simulink model "modelR2020a"  (R2020a)
settings: Solver=ode23s  StartTime=0.0  StopTime=settings.Tsim  FixedStep=0.1  RelTol=1e-6  AbsTol=1e-6
values from neighbouring files (symbols this model uses):
  settings = Simulink.Parameter    [main.m]
libraries: vrlib x5
settings Model: Creator=rosat  LastModifiedBy=rosat
settings SolverCC: ZeroCrossAlgorithm=Adaptive
settings OptimizationCC: BlockReduction=off  DefaultParameterBehavior=Inlined  BufferReuse=off
settings DebuggingCC: IgnoredZcDiagnostic=none  SFMachineParentedDataDiag=error

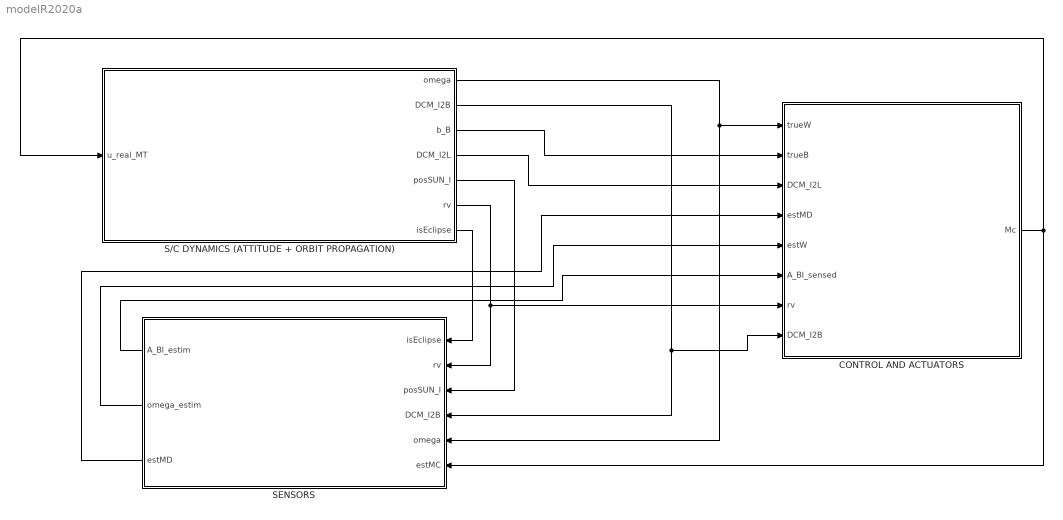
== system modelR2020a ==
  CONTROL AND ACTUATORS : Subsystem
  S/C DYNAMICS (ATTITUDE + ORBIT PROPAGATION) : Subsystem
  SENSORS : Subsystem
  wires:
  S/C DYNAMICS (ATTITUDE + ORBIT PROPAGATION)/3(b_B) -> CONTROL AND ACTUATORS/2(trueB)
  SENSORS/1(A_BI_estim) -> CONTROL AND ACTUATORS/6(A_BI_sensed)
  S/C DYNAMICS (ATTITUDE + ORBIT PROPAGATION)/6(rv) -> CONTROL AND ACTUATORS/7(rv), SENSORS/2(rv)
  SENSORS/3(estMD) -> CONTROL AND ACTUATORS/4(estMD)
  SENSORS/2(omega_estim) -> CONTROL AND ACTUATORS/5(estW)
  S/C DYNAMICS (ATTITUDE + ORBIT PROPAGATION)/2(DCM_I2B) -> CONTROL AND ACTUATORS/8(DCM_I2B), SENSORS/4(DCM_I2B)
  S/C DYNAMICS (ATTITUDE + ORBIT PROPAGATION)/1(omega) -> CONTROL AND ACTUATORS/1(trueW), SENSORS/5(omega)
  S/C DYNAMICS (ATTITUDE + ORBIT PROPAGATION)/4(DCM_I2L) -> CONTROL AND ACTUATORS/3(DCM_I2L)
  S/C DYNAMICS (ATTITUDE + ORBIT PROPAGATION)/5(posSUN_I) -> SENSORS/3(posSUN_I)
  CONTROL AND ACTUATORS/1(Mc) -> S/C DYNAMICS (ATTITUDE + ORBIT PROPAGATION)/1(u_real_MT), SENSORS/6(estMC)
  S/C DYNAMICS (ATTITUDE + ORBIT PROPAGATION)/7(isEclipse) -> SENSORS/1(isEclipse)

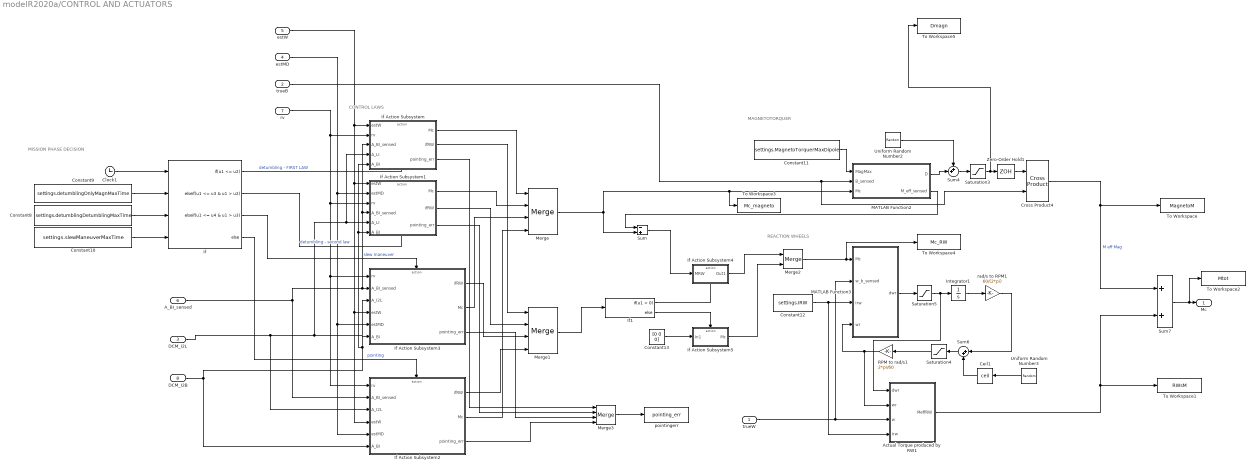
== system modelR2020a/CONTROL AND ACTUATORS ==
  note: REACTION WHEELS
  note: CONTROL LAWS
  note: MISSION PHASE DECISION
  note: MAGNETOTORQUER
  trueW : Inport
  trueB : Inport  Port=2
  DCM_I2L : Inport  Port=3
  estMD : Inport  Port=4
  estW : Inport  Port=5
  A_BI_sensed : Inport  Port=6
  rv : Inport  Port=7
  DCM_I2B : Inport  Port=8
  Actual Torque produced by RW1 : MATLAB Function  TreatAsAtomicUnit=on
  Ceil1 : Rounding  Operator=ceil
  Clock1 : Clock
  Constant10 : Constant  Value=settings.slewManeuverMaxTime
  Constant11 : Constant  Value=settings.MagnetoTorquerMaxDipole
  Constant12 : Constant  Value=settings.IRW
  Constant13 : Constant  Value=[0 0 0]
  Constant8 : Constant  Value=settings.detumblingDetumblingMaxTime
  Constant9 : Constant  Value=settings.detumblingOnlyMagnMaxTime
  Cross Product4 : vrlib/Utilities/Cross Product
  If : If  NumInputs=4  IfExpression=u1 <= u2  ElseIfExpressions=u1 <= u3 & u1 > u2, u1 <= u4 & u1 > u3
  If Action Subsystem : Subsystem  TreatAsAtomicUnit=on
  If Action Subsystem1 : Subsystem  TreatAsAtomicUnit=on
  If Action Subsystem2 : Subsystem  TreatAsAtomicUnit=on
  If Action Subsystem3 : Subsystem  TreatAsAtomicUnit=on
  If Action Subsystem4 : Subsystem  TreatAsAtomicUnit=on
  If Action Subsystem5 : Subsystem  TreatAsAtomicUnit=on
  If1 : If
  Integrator1 : Integrator  InitialCondition=[0;0;0]
  MATLAB Function2 : MATLAB Function  TreatAsAtomicUnit=on
  MATLAB Function3 : MATLAB Function  TreatAsAtomicUnit=on
  Merge : Merge  Inputs=4
  Merge1 : Merge  Inputs=4
  Merge2 : Merge
  Merge3 : Merge  Inputs=4
  RPM to rad/s1 : Gain  Gain=2*pi/60
  Saturation3 : Saturate  UpperLimit=settings.MagnetoTorquerMaxDipole  LowerLimit=-settings.MagnetoTorquerMaxDipole
  Saturation4 : Saturate  UpperLimit=settings.MaxRPM*[1;1;1]  LowerLimit=-settings.MaxRPM*[1;1;1]  LinearizeAsGain=off  ZeroCross=off
  Saturation5 : Saturate  UpperLimit=settings.MaxRPM_Rate  LowerLimit=-settings.MaxRPM_Rate
  Sum : Sum  Inputs=-+
  Sum4 : Sum  Inputs=++|
  Sum6 : Sum  Inputs=|++
  Sum7 : Sum
  To Workspace : ToWorkspace  VariableName=MagnetoM  SaveFormat=Timeseries  SampleTime=-1
  To Workspace1 : ToWorkspace  VariableName=RWsM  SaveFormat=Timeseries  SampleTime=-1
  To Workspace2 : ToWorkspace  VariableName=Mtot  SaveFormat=Timeseries  SampleTime=-1
  To Workspace3 : ToWorkspace  VariableName=Mc_magneto  SaveFormat=Timeseries  SampleTime=-1
  To Workspace4 : ToWorkspace  VariableName=Mc_RW  SaveFormat=Timeseries  SampleTime=-1
  To Workspace5 : ToWorkspace  VariableName=Dmagn  SaveFormat=Timeseries  SampleTime=-1
  Uniform Random Number2 : UniformRandomNumber  Minimum=-settings.MagnetoTorquerDipoleError*[1;1;1]  Maximum=settings.MagnetoTorquerDipoleError*[1;1;1]  Seed=456156  SampleTime=1/settings.MagnetoTorquerSampleRate
  Uniform Random Number3 : UniformRandomNumber  Minimum=-settings.RPMAccuracy*[1;1;1]  Maximum=settings.RPMAccuracy*[1;1;1]  Seed=561651  SampleTime=1/settings.RW_sr
  Zero-Order Hold1 : ZeroOrderHold  SampleTime=1/settings.MagnetoTorquerSampleRate
  pointingerr : ToWorkspace  VariableName=pointing_err  SaveFormat=Timeseries  SampleTime=-1
  rad/s to RPM1 : Gain  Gain=60/(2*pi)
  Mc : Outport
  wires:
  Clock1/1 -> If/1
  Constant9/1 -> If/2
  Constant8/1 -> If/3
  If/1 -> If Action Subsystem/Action  "detumbling - FIRST LAW"
  If/2 -> If Action Subsystem1/Action  "detumbling - second law"
  If/4 -> If Action Subsystem2/Action  "pointing"
  Constant10/1 -> If/4
  If/3 -> If Action Subsystem3/Action  "slew maneuver"
  Sum4/1 -> Saturation3/1
  Zero-Order Hold1/1 -> Cross Product4/1
  Constant11/1 -> MATLAB Function2/1(MagMax)
  Saturation3/1 -> To Workspace5/1, Zero-Order Hold1/1
  Uniform Random Number2/1 -> Sum4/1
  If Action Subsystem/1(Mc) -> Merge/1
  If Action Subsystem1/1(Mc) -> Merge/2
  If Action Subsystem/2(ifRW) -> Merge1/1
  If Action Subsystem1/2(ifRW) -> Merge1/2
  If Action Subsystem3/2(Mc) -> Merge/3
  If Action Subsystem3/1(ifRW) -> Merge1/3
  Cross Product4/1 -> To Workspace/1, Sum7/1  "M eff Mag"
  rad/s to RPM1/1 -> Sum6/1
  Uniform Random Number3/1 -> Ceil1/1
  RPM to rad/s1/1 -> Actual Torque produced by RW1/2(wr), MATLAB Function3/4(wr)
  Constant12/1 -> Actual Torque produced by RW1/4(Irw), MATLAB Function3/3(Irw)
  MATLAB Function3/1(dwr) -> Saturation5/1
  Saturation4/1 -> RPM to rad/s1/1
  Sum6/1 -> Saturation4/1
  Integrator1/1 -> rad/s to RPM1/1
  Saturation5/1 -> Actual Torque produced by RW1/1(dwr), Integrator1/1
  If1/1 -> If Action Subsystem4/Action
  If1/2 -> If Action Subsystem5/Action
  Constant13/1 -> If Action Subsystem5/1(In1)
  Merge2/1 -> To Workspace4/1, MATLAB Function3/1(Mc)
  If Action Subsystem4/1(Out1) -> Merge2/1
  If Action Subsystem5/1(Mc) -> Merge2/2
  Sum7/1 -> To Workspace2/1, Mc/1
  Actual Torque produced by RW1/1(MeffRW) -> To Workspace1/1, Sum7/2
  MATLAB Function2/1(D) -> Sum4/2
  Merge1/1 -> If1/1
  Sum/1 -> If Action Subsystem4/1(MRW)
  Ceil1/1 -> Sum6/2
  MATLAB Function2/2(M_eff_sensed) -> Sum/1
  Merge/1 -> To Workspace3/1, MATLAB Function2/3(Mc), Sum/2
  estW/1 -> If Action Subsystem2/4(estW), If Action Subsystem3/4(estW), If Action Subsystem1/1(estW), If Action Subsystem/1(estW)
  trueW/1 -> Actual Torque produced by RW1/3(w), MATLAB Function3/2(w_b_sensed)
  estMD/1 -> If Action Subsystem2/5(estMD), If Action Subsystem3/5(estMD), If Action Subsystem1/2(estMD)
  trueB/1 -> Cross Product4/2, MATLAB Function2/2(B_sensed)
  rv/1 -> If Action Subsystem/2(rv), If Action Subsystem1/3(rv), If Action Subsystem2/1(rv), If Action Subsystem3/1(rv)
  A_BI_sensed/1 -> If Action Subsystem1/4(A_BI_sensed), If Action Subsystem/3(A_BI_sensed), If Action Subsystem3/2(A_BI_sensed), If Action Subsystem2/2(A_BI_sensed)
  DCM_I2B/1 -> If Action Subsystem1/6(A_BI), If Action Subsystem/5(A_BI), If Action Subsystem3/6(A_BI), If Action Subsystem2/6(A_BI)
  DCM_I2L/1 -> If Action Subsystem3/3(A_I2L), If Action Subsystem1/5(A_LI), If Action Subsystem/4(A_LI), If Action Subsystem2/3(A_I2L)
  If Action Subsystem2/2(Mc) -> Merge/4
  If Action Subsystem2/1(ifRW) -> Merge1/4
  If Action Subsystem/3(pointing_err) -> Merge3/1
  If Action Subsystem1/3(pointing_err) -> Merge3/2
  If Action Subsystem3/3(pointing_err) -> Merge3/3
  If Action Subsystem2/3(pointing_err) -> Merge3/4
  Merge3/1 -> pointingerr/1

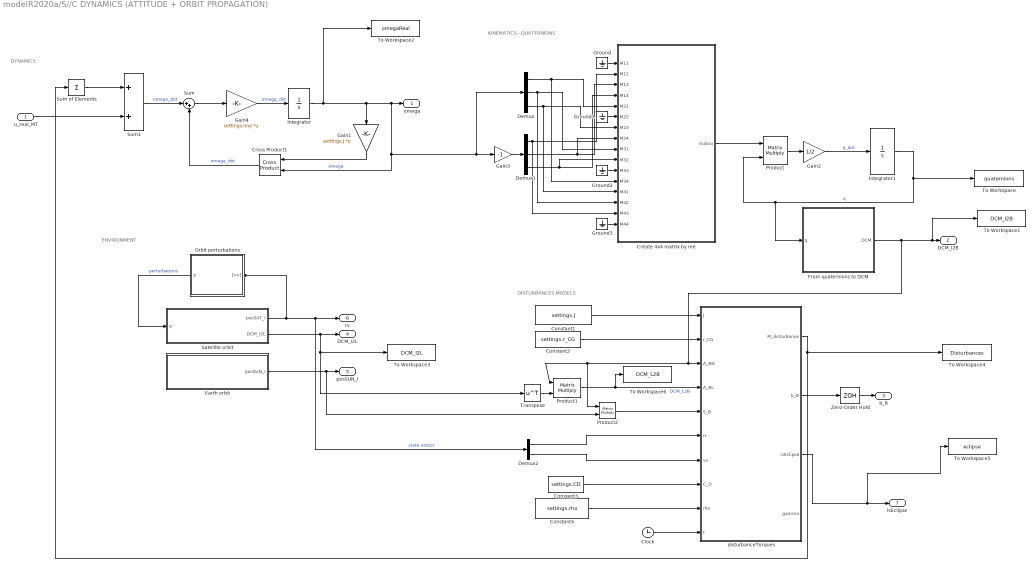
== system modelR2020a/S//C DYNAMICS (ATTITUDE + ORBIT PROPAGATION) ==
  note: DISTURBANCES MODELS
  note: ENVIRONMENT
  note: KINEMATICS - QUATERNIONS
  note: DYNAMICS
  u_real_MT : Inport
  Clock : Clock
  Constant1 : Constant  Value=settings.J
  Constant2 : Constant  Value=settings.r_CG
  Constant3 : Constant  Value=settings.CD
  Constant4 : Constant  Value=settings.rho
  Create 4x4 matrix by me : Subsystem
  Cross Product1 : vrlib/Utilities/Cross Product
  Demux : Demux  Outputs=3
  Demux1 : Demux  Outputs=3
  Demux2 : Demux  Outputs=2
  Earth orbit : Subsystem
  From quaternions to DCM : Subsystem
  Gain1 : Gain  Gain=settings.J  Multiplication=Matrix(K*u)
  Gain2 : Gain  Gain=1/2
  Gain3 : Gain  Gain=-1
  Gain4 : Gain  Gain=settings.invJ  Multiplication=Matrix(K*u)
  Ground{,1..3} (4 alike) : Ground
  Integrator : Integrator  InitialCondition=settings.omega0
  Integrator1 : Integrator  InitialCondition=settings.q0
  Orbit perturbations : Subsystem
  Product : Product  Multiplication=Matrix(*)
  Product1 : Product  Multiplication=Matrix(*)
  Product2 : Product  Multiplication=Matrix(*)
  Satellite orbit : Subsystem
  Sum : Sum  Inputs=|++
  Sum of Elements : Sum  Inputs=+  CollapseMode=Specified dimension  CollapseDim=2
  Sum1 : Sum
  To Workspace : ToWorkspace  VariableName=quaternions  SaveFormat=Timeseries  SampleTime=-1
  To Workspace1 : ToWorkspace  VariableName=DCM_I2B  SaveFormat=Timeseries  SampleTime=-1
  To Workspace2 : ToWorkspace  VariableName=omegaReal  SaveFormat=Timeseries  SampleTime=-1
  To Workspace3 : ToWorkspace  VariableName=DCM_I2L  SaveFormat=Timeseries  SampleTime=-1
  To Workspace4 : ToWorkspace  VariableName=Disturbances  SaveFormat=Timeseries  SampleTime=-1
  To Workspace5 : ToWorkspace  VariableName=eclipse  SaveFormat=Timeseries  SampleTime=-1
  To Workspace6 : ToWorkspace  VariableName=DCM_L2B  SaveFormat=Timeseries  SampleTime=-1
  Transpose : Math  Operator=transpose  SaturateOnIntegerOverflow=on
  Zero-Order Hold : ZeroOrderHold  SampleTime=0.01
  disturbanceTorques : MATLAB Function  TreatAsAtomicUnit=on
  omega : Outport
  DCM_I2B : Outport  Port=2
  b_B : Outport  Port=3
  DCM_I2L : Outport  Port=4
  posSUN_I : Outport  Port=5
  rv : Outport  Port=6
  isEclipse : Outport  Port=7
  wires:
  Sum of Elements/1 -> Sum1/1
  Integrator/1 -> Demux/1, Gain3/1, Cross Product1/2, omega/1, Gain1/1, To Workspace2/1  "omega"
  Sum/1 -> Gain4/1
  u_real_MT/1 -> Sum1/2
  Sum1/1 -> Sum/1  "omega_dot"
  Gain4/1 -> Integrator/1  "omega_dot"
  Cross Product1/1 -> Sum/2  "omega_dot"
  Gain1/1 -> Cross Product1/1
  disturbanceTorques/1(M_disturbance) -> To Workspace4/1, Sum of Elements/1
  Demux/3 -> Create 4x4 matrix by me/13(M41), Create 4x4 matrix by me/7(M23)
  Product/1 -> Gain2/1
  Demux1/2 -> Create 4x4 matrix by me/8(M24), Create 4x4 matrix by me/3(M13)
  Demux1/3 -> Create 4x4 matrix by me/10(M32), Create 4x4 matrix by me/4(M14)
  Demux1/1 -> Create 4x4 matrix by me/15(M43), Create 4x4 matrix by me/2(M12)
  Demux/1 -> Create 4x4 matrix by me/12(M34), Create 4x4 matrix by me/5(M21)
  Ground2/1 -> Create 4x4 matrix by me/11(M33)
  Ground/1 -> Create 4x4 matrix by me/1(M11)
  From quaternions to DCM/1(DCM) -> Product2/1, Product1/1, disturbanceTorques/3(A_BN), To Workspace1/1, DCM_I2B/1
  Demux/2 -> Create 4x4 matrix by me/14(M42), Create 4x4 matrix by me/9(M31)
  Ground3/1 -> Create 4x4 matrix by me/16(M44)
  Gain2/1 -> Integrator1/1  "q_dot"
  Integrator1/1 -> To Workspace/1, From quaternions to DCM/1(q), Product/2  "q"
  Gain3/1 -> Demux1/1
  Ground1/1 -> Create 4x4 matrix by me/6(M22)
  Create 4x4 matrix by me/1(matrix) -> Product/1
  Earth orbit/1(posSUN_I) -> Product2/2, posSUN_I/1
  Satellite orbit/1(posSAT_I) -> Orbit perturbations/1("[r;v]"), Demux2/1, rv/1  "state vector"
  Orbit perturbations/1(p) -> Satellite orbit/1(p)  "perturbations"
  Satellite orbit/2(DCM_I2L) -> Transpose/1, To Workspace3/1, DCM_I2L/1
  Constant3/1 -> disturbanceTorques/8(C_D)
  Constant2/1 -> disturbanceTorques/2(r_CG)
  Demux2/2 -> disturbanceTorques/7(vv)
  Demux2/1 -> disturbanceTorques/6(rr)
  Constant4/1 -> disturbanceTorques/9(rho)
  Clock/1 -> disturbanceTorques/10(t)
  Transpose/1 -> Product1/2
  Product2/1 -> disturbanceTorques/5(S_B)
  Product1/1 -> To Workspace6/1, disturbanceTorques/4(A_BL)  "DCM_L2B"
  Constant1/1 -> disturbanceTorques/1(J)
  disturbanceTorques/2(b_B) -> Zero-Order Hold/1
  Zero-Order Hold/1 -> b_B/1
  disturbanceTorques/3(isEclipse) -> To Workspace5/1, isEclipse/1

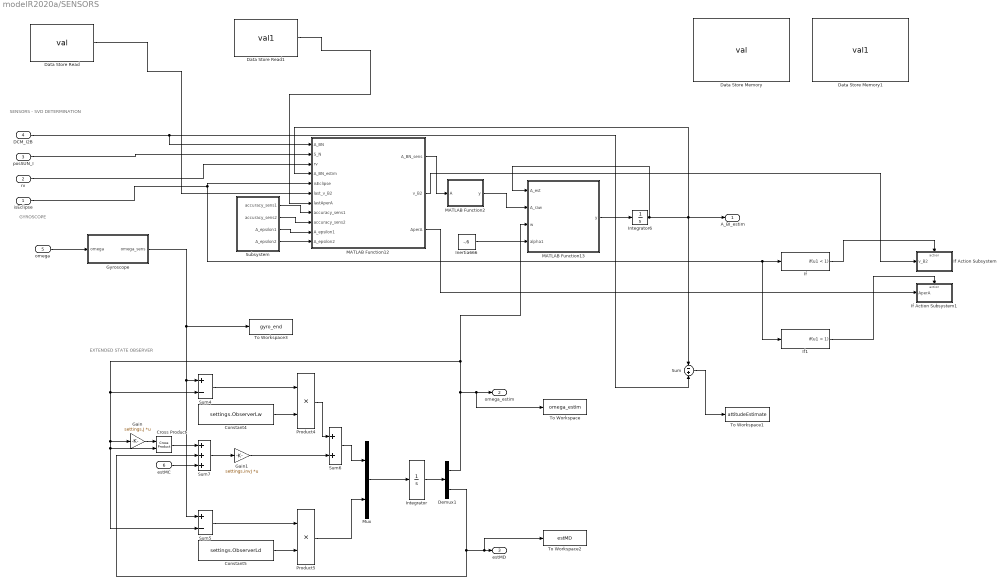
== system modelR2020a/SENSORS ==
  note: GYROSCOPE
  note: EXTENDED STATE OBSERVER
  note: SENSORS - SVD DETERMINATION
  isEclipse : Inport
  rv : Inport  Port=2
  posSUN_I : Inport  Port=3
  DCM_I2B : Inport  Port=4
  omega : Inport  Port=5
  estMC : Inport  Port=6
  Constant4 : Constant  Value=settings.ObserverLw
  Constant5 : Constant  Value=settings.ObserverLd
  Cross Product : vrlib/Utilities/Cross Product
  Data Store Memory : DataStoreMemory  DataStoreName=val  ReadBeforeWriteMsg=warning  WriteAfterWriteMsg=warning  WriteAfterReadMsg=warning  VectorParams1D=off  ShowAdditionalParam=off  Dimensions=3
  Data Store Memory1 : DataStoreMemory  DataStoreName=val1  ReadBeforeWriteMsg=warning  WriteAfterWriteMsg=warning  WriteAfterReadMsg=warning  VectorParams1D=off  ShowAdditionalParam=off  Dimensions=[3,3]
  Data Store Read : DataStoreRead  DataStoreName=val
  Data Store Read1 : DataStoreRead  DataStoreName=val1
  Demux1 : Demux  Outputs=2
  Gain : Gain  Gain=settings.J  Multiplication=Matrix(K*u)
  Gain1 : Gain  Gain=settings.invJ  Multiplication=Matrix(K*u)
  Gyroscope : Subsystem
  If : If  IfExpression=u1 < 1  ShowElse=off
  If Action Subsystem : Subsystem  TreatAsAtomicUnit=on
  If Action Subsystem1 : Subsystem  TreatAsAtomicUnit=on
  If1 : If  IfExpression=u1 < 1  ShowElse=off
  Inertia666 : Constant  Value=-.6
  Integrator : Integrator  InitialCondition=[settings.omega0; settings.ObserverMd0]
  Integrator6 : Integrator  InitialCondition=zeros(3,3)
  MATLAB Function12 : MATLAB Function  TreatAsAtomicUnit=on
  MATLAB Function13 : MATLAB Function  TreatAsAtomicUnit=on
  MATLAB Function2 : MATLAB Function  TreatAsAtomicUnit=on
  Mux : Mux  Inputs=2
  Product4 : Product
  Product5 : Product
  Subsystem : Subsystem
  Sum : Sum  Inputs=-+
  Sum4 : Sum  Inputs=+-
  Sum5 : Sum  Inputs=+-
  Sum6 : Sum
  Sum7 : Sum  Inputs=+++
  To Workspace : ToWorkspace  VariableName=omega_estim  SaveFormat=Timeseries  SampleTime=-1
  To Workspace1 : ToWorkspace  VariableName=attitudeEstimate  SaveFormat=Timeseries  SampleTime=-1
  To Workspace2 : ToWorkspace  VariableName=estMD  SaveFormat=Timeseries  SampleTime=-1
  To Workspace3 : ToWorkspace  VariableName=gyro_end  SaveFormat=Timeseries  SampleTime=-1
  A_BI_estim : Outport
  omega_estim : Outport  Port=2
  estMD : Outport  Port=3
  wires:
  DCM_I2B/1 -> Sum/2, MATLAB Function12/1(A_BN)
  posSUN_I/1 -> MATLAB Function12/2(S_N)
  omega/1 -> Gyroscope/1(omega)
  Gyroscope/1(omega_sens) -> To Workspace3/1, Sum5/1, Sum4/1
  Sum4/1 -> Product4/1
  Constant4/1 -> Product4/2
  Constant5/1 -> Product5/2
  Sum5/1 -> Product5/1
  Integrator/1 -> Demux1/1
  Demux1/1 -> MATLAB Function13/3(w), Sum5/2, Cross Product/2, Gain/1, Sum4/2, To Workspace/1, omega_estim/1
  Product4/1 -> Sum6/1
  Gain/1 -> Cross Product/1
  Cross Product/1 -> Sum7/1
  Demux1/2 -> To Workspace2/1, estMD/1, Sum7/2
  Sum7/1 -> Gain1/1
  Gain1/1 -> Sum6/2
  Sum6/1 -> Mux/1
  Product5/1 -> Mux/2
  Mux/1 -> Integrator/1
  estMC/1 -> Sum7/3
  Subsystem/1(accuracy_sens1) -> MATLAB Function12/8(accuracy_sens1)
  Subsystem/4(A_epsilon2) -> MATLAB Function12/11(A_epsilon2)
  MATLAB Function13/1(y) -> Integrator6/1
  MATLAB Function12/1(A_BN_sens) -> MATLAB Function2/1(A)
  Subsystem/3(A_epsilon1) -> MATLAB Function12/10(A_epsilon1)
  MATLAB Function2/1(y) -> MATLAB Function13/2(A_raw)
  Inertia666/1 -> MATLAB Function13/4(alpha1)
  Subsystem/2(accuracy_sens2) -> MATLAB Function12/9(accuracy_sens2)
  rv/1 -> MATLAB Function12/3(rv)
  Integrator6/1 -> A_BI_estim/1, MATLAB Function12/4(A_BN_estim), Sum/1, MATLAB Function13/1(A_est)
  isEclipse/1 -> If1/1, If/1, MATLAB Function12/5(isEclipse)
  MATLAB Function12/2(v_B2) -> If Action Subsystem/1(v_B2)
  If/1 -> If Action Subsystem/Action
  Data Store Read/1 -> MATLAB Function12/6(last_v_B2)
  MATLAB Function12/3(AperA) -> If Action Subsystem1/1(AperA)
  Data Store Read1/1 -> MATLAB Function12/7(lastAperA)
  If1/1 -> If Action Subsystem1/Action
  Sum/1 -> To Workspace1/1

== system modelR2020a/CONTROL AND ACTUATORS/If Action Subsystem ==
  estW : Inport
  rv : Inport  Port=2
  A_BI_sensed : Inport  Port=3
  A_LI : Inport  Port=4
  A_BI : Inport  Port=5
  Action Port : ActionPort  ActionPortLabel=if(u1 <= u2)
  Constant : Constant  Value=settings.detumblingkb
  Constant1 : Constant  Value=0
  Gain : Gain  Gain=-1
  MATLAB Function : MATLAB Function  TreatAsAtomicUnit=on
  Product : Product
  Mc : Outport
  ifRW : Outport  Port=2
  pointing_err : Outport  Port=3
  wires:
  Constant/1 -> Product/2
  Constant1/1 -> ifRW/1
  Product/1 -> Gain/1
  Gain/1 -> Mc/1
  A_BI_sensed/1 -> MATLAB Function/2(A_BI_sensed)
  MATLAB Function/3(pointing_err) -> pointing_err/1
  estW/1 -> MATLAB Function/4(estW), Product/1
  A_LI/1 -> MATLAB Function/3(A_LI)
  rv/1 -> MATLAB Function/1(rv)
  A_BI/1 -> MATLAB Function/5(A_BI)

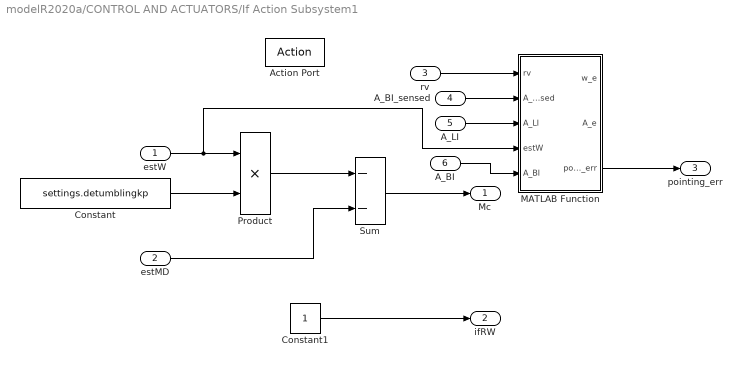
== system modelR2020a/CONTROL AND ACTUATORS/If Action Subsystem1 ==
  estW : Inport
  estMD : Inport  Port=2
  rv : Inport  Port=3
  A_BI_sensed : Inport  Port=4
  A_LI : Inport  Port=5
  A_BI : Inport  Port=6
  Action Port : ActionPort  ActionPortLabel=elseif(u1 <= u3 & u1 > u2)
  Constant : Constant  Value=settings.detumblingkp
  Constant1 : Constant
  MATLAB Function : MATLAB Function  TreatAsAtomicUnit=on
  Product : Product
  Sum : Sum  Inputs=--
  Mc : Outport
  ifRW : Outport  Port=2
  pointing_err : Outport  Port=3
  wires:
  estW/1 -> MATLAB Function/4(estW), Product/1
  Constant/1 -> Product/2
  Product/1 -> Sum/1
  estMD/1 -> Sum/2
  Sum/1 -> Mc/1
  Constant1/1 -> ifRW/1
  MATLAB Function/3(pointing_err) -> pointing_err/1
  rv/1 -> MATLAB Function/1(rv)
  A_BI_sensed/1 -> MATLAB Function/2(A_BI_sensed)
  A_LI/1 -> MATLAB Function/3(A_LI)
  A_BI/1 -> MATLAB Function/5(A_BI)

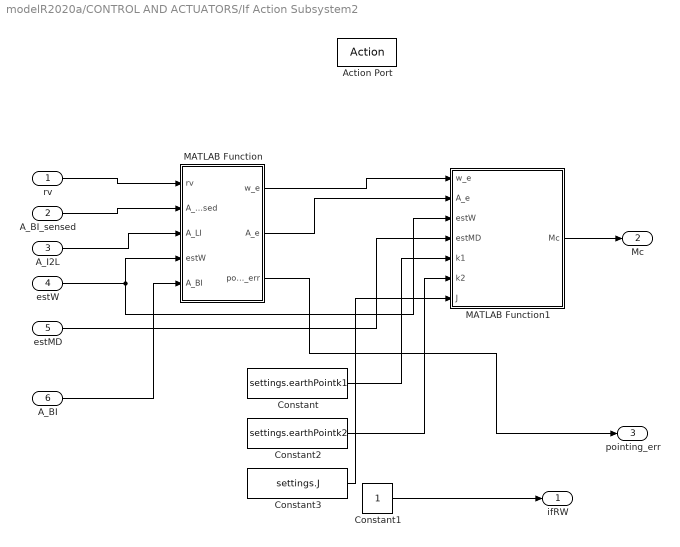
== system modelR2020a/CONTROL AND ACTUATORS/If Action Subsystem2 ==
  rv : Inport
  A_BI_sensed : Inport  Port=2
  A_I2L : Inport  Port=3
  estW : Inport  Port=4
  estMD : Inport  Port=5
  A_BI : Inport  Port=6
  Action Port : ActionPort  ActionPortLabel=else
  Constant : Constant  Value=settings.earthPointk1
  Constant1 : Constant
  Constant2 : Constant  Value=settings.earthPointk2
  Constant3 : Constant  Value=settings.J
  MATLAB Function : MATLAB Function  TreatAsAtomicUnit=on
  MATLAB Function1 : MATLAB Function  TreatAsAtomicUnit=on
  ifRW : Outport
  Mc : Outport  Port=2
  pointing_err : Outport  Port=3
  wires:
  A_BI/1 -> MATLAB Function/5(A_BI)
  estMD/1 -> MATLAB Function1/4(estMD)
  MATLAB Function/3(pointing_err) -> pointing_err/1
  rv/1 -> MATLAB Function/1(rv)
  Constant3/1 -> MATLAB Function1/7(J)
  A_BI_sensed/1 -> MATLAB Function/2(A_BI_sensed)
  A_I2L/1 -> MATLAB Function/3(A_LI)
  Constant2/1 -> MATLAB Function1/6(k2)
  estW/1 -> MATLAB Function1/3(estW), MATLAB Function/4(estW)
  Constant1/1 -> ifRW/1
  MATLAB Function1/1(Mc) -> Mc/1
  Constant/1 -> MATLAB Function1/5(k1)
  MATLAB Function/1(w_e) -> MATLAB Function1/1(w_e)
  MATLAB Function/2(A_e) -> MATLAB Function1/2(A_e)

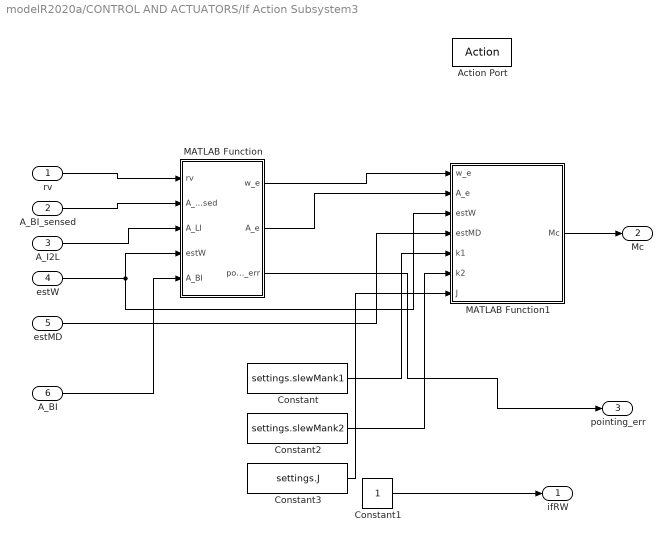
== system modelR2020a/CONTROL AND ACTUATORS/If Action Subsystem3 ==
  rv : Inport
  A_BI_sensed : Inport  Port=2
  A_I2L : Inport  Port=3
  estW : Inport  Port=4
  estMD : Inport  Port=5
  A_BI : Inport  Port=6
  Action Port : ActionPort  ActionPortLabel=elseif( u1 <= u4 & u1 > u3)
  Constant : Constant  Value=settings.slewMank1
  Constant1 : Constant
  Constant2 : Constant  Value=settings.slewMank2
  Constant3 : Constant  Value=settings.J
  MATLAB Function : MATLAB Function  TreatAsAtomicUnit=on
  MATLAB Function1 : MATLAB Function  TreatAsAtomicUnit=on
  ifRW : Outport
  Mc : Outport  Port=2
  pointing_err : Outport  Port=3
  wires:
  Constant1/1 -> ifRW/1
  rv/1 -> MATLAB Function/1(rv)
  estW/1 -> MATLAB Function1/3(estW), MATLAB Function/4(estW)
  A_I2L/1 -> MATLAB Function/3(A_LI)
  A_BI_sensed/1 -> MATLAB Function/2(A_BI_sensed)
  estMD/1 -> MATLAB Function1/4(estMD)
  MATLAB Function/1(w_e) -> MATLAB Function1/1(w_e)
  MATLAB Function/2(A_e) -> MATLAB Function1/2(A_e)
  MATLAB Function1/1(Mc) -> Mc/1
  Constant/1 -> MATLAB Function1/5(k1)
  Constant2/1 -> MATLAB Function1/6(k2)
  Constant3/1 -> MATLAB Function1/7(J)
  A_BI/1 -> MATLAB Function/5(A_BI)
  MATLAB Function/3(pointing_err) -> pointing_err/1

== system modelR2020a/CONTROL AND ACTUATORS/If Action Subsystem4 ==
  MRW : Inport
  Action Port : ActionPort  ActionPortLabel=if(u1 > 0)
  Out1 : Outport
  wires:
  MRW/1 -> Out1/1

== system modelR2020a/CONTROL AND ACTUATORS/If Action Subsystem5 ==
  In1 : Inport
  Action Port : ActionPort  ActionPortLabel=else
  Mc : Outport
  wires:
  In1/1 -> Mc/1

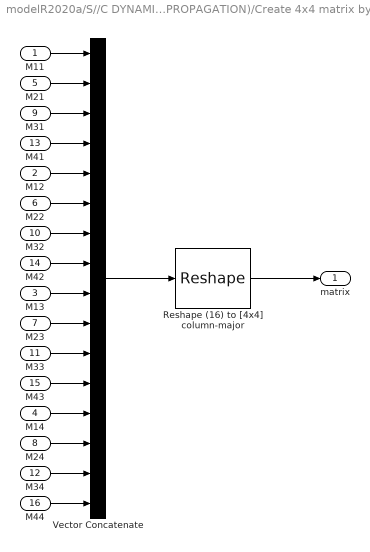
== system modelR2020a/S//C DYNAMICS (ATTITUDE + ORBIT PROPAGATION)/Create 4x4 matrix by me ==
  M11 : Inport
  M12 : Inport  Port=2
  M13 : Inport  Port=3
  M14 : Inport  Port=4
  M21 : Inport  Port=5
  M22 : Inport  Port=6
  M23 : Inport  Port=7
  M24 : Inport  Port=8
  M31 : Inport  Port=9
  M32 : Inport  Port=10
  M33 : Inport  Port=11
  M34 : Inport  Port=12
  M41 : Inport  Port=13
  M42 : Inport  Port=14
  M43 : Inport  Port=15
  M44 : Inport  Port=16
  Reshape (16) to [4x4] column-major : Reshape  OutputDimensionality=Customize  OutputDimensions=[4,4]
  Vector Concatenate : Concatenate  NumInputs=16
  matrix : Outport
  wires:
  M12/1 -> Vector Concatenate/5
  M11/1 -> Vector Concatenate/1
  M13/1 -> Vector Concatenate/9
  M14/1 -> Vector Concatenate/13
  M21/1 -> Vector Concatenate/2
  M44/1 -> Vector Concatenate/16
  M34/1 -> Vector Concatenate/15
  M24/1 -> Vector Concatenate/14
  M43/1 -> Vector Concatenate/12
  M33/1 -> Vector Concatenate/11
  M23/1 -> Vector Concatenate/10
  M42/1 -> Vector Concatenate/8
  M32/1 -> Vector Concatenate/7
  M22/1 -> Vector Concatenate/6
  M41/1 -> Vector Concatenate/4
  M31/1 -> Vector Concatenate/3
  Vector Concatenate/1 -> Reshape (16) to [4x4] column-major/1
  Reshape (16) to [4x4] column-major/1 -> matrix/1

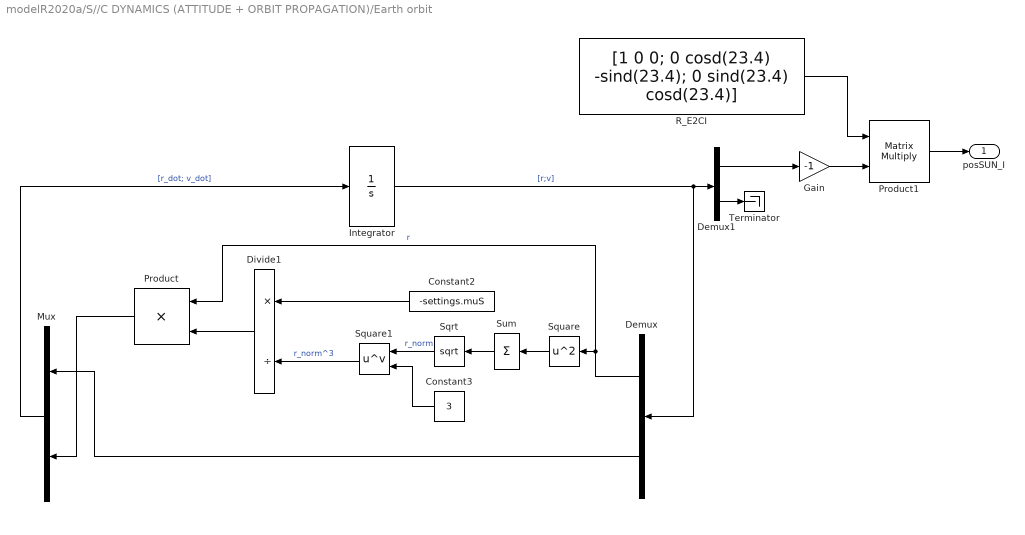
== system modelR2020a/S//C DYNAMICS (ATTITUDE + ORBIT PROPAGATION)/Earth orbit ==
  Constant2 : Constant  Value=-settings.muS
  Constant3 : Constant  Value=3
  Demux : Demux  Outputs=2
  Demux1 : Demux  Outputs=2
  Divide1 : Product  Inputs=*/
  Gain : Gain  Gain=-1
  Integrator : Integrator  InitialCondition=settings.Y0E
  Mux : Mux  Inputs=2
  Product : Product
  Product1 : Product  Multiplication=Matrix(*)
  R_E2CI : Constant  Value=[1 0 0; 0 cosd(23.4) -sind(23.4); 0 sind(23.4) cosd(23.4)]  VectorParams1D=off
  Sqrt : Sqrt  SaturateOnIntegerOverflow=on
  Square : Math  Operator=square  SaturateOnIntegerOverflow=on
  Square1 : Math  Operator=pow  SaturateOnIntegerOverflow=on
  Sum : Sum  Inputs=+
  Terminator : Terminator
  posSUN_I : Outport
  wires:
  Constant3/1 -> Square1/2
  Demux/1 -> Product/1, Square/1  "r"
  Demux/2 -> Mux/1
  Integrator/1 -> Demux1/1, Demux/1  "[r;v]"
  Divide1/1 -> Product/2
  Sqrt/1 -> Square1/1  "r_norm"
  Constant2/1 -> Divide1/1
  Product/1 -> Mux/2
  Sum/1 -> Sqrt/1
  Square/1 -> Sum/1
  Square1/1 -> Divide1/2  "r_norm^3"
  Mux/1 -> Integrator/1  "[r_dot; v_dot]"
  Gain/1 -> Product1/2
  R_E2CI/1 -> Product1/1
  Demux1/1 -> Gain/1
  Demux1/2 -> Terminator/1
  Product1/1 -> posSUN_I/1

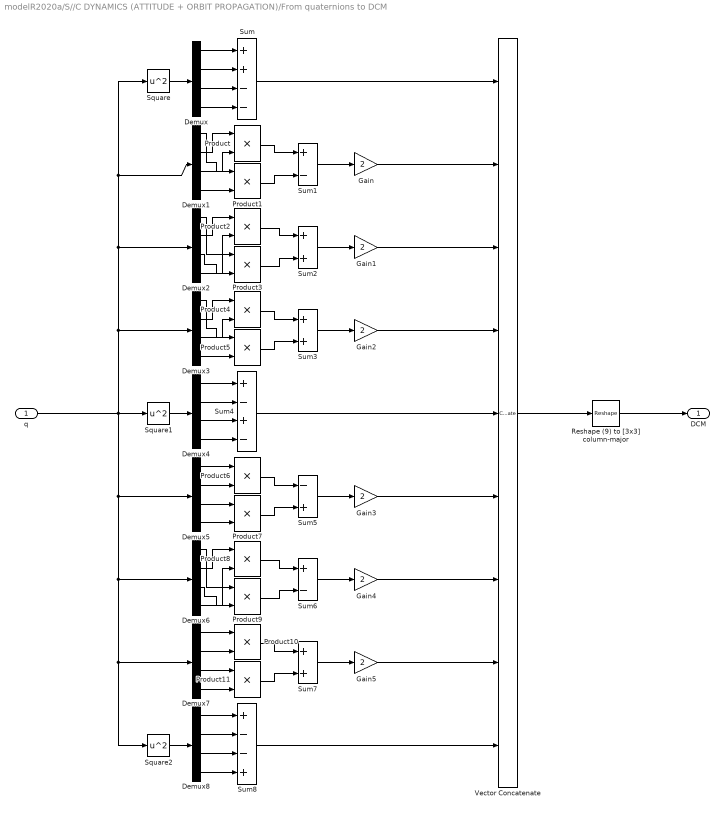
== system modelR2020a/S//C DYNAMICS (ATTITUDE + ORBIT PROPAGATION)/From quaternions to DCM ==
  q : Inport
  Demux{,1..8} (9 alike) : Demux
  Gain{,1..5} (6 alike) : Gain  Gain=2
  Product{,1..11} (12 alike) : Product
  Reshape (9) to [3x3] column-major : Reshape  OutputDimensionality=Customize  OutputDimensions=[3,3]
  Square : Math  Operator=square  SaturateOnIntegerOverflow=on
  Square1 : Math  Operator=square  SaturateOnIntegerOverflow=on
  Square2 : Math  Operator=square  SaturateOnIntegerOverflow=on
  Sum : Sum  Inputs=++--
  Sum1 : Sum  Inputs=+-
  Sum2 : Sum
  Sum3 : Sum
  Sum4 : Sum  Inputs=+-+-
  Sum5 : Sum  Inputs=-+
  Sum6 : Sum  Inputs=+-
  Sum7 : Sum
  Sum8 : Sum  Inputs=+--+
  Vector Concatenate : Concatenate  NumInputs=9
  DCM : Outport
  wires:
  q/1 -> Square/1, Demux1/1, Demux2/1, Demux3/1, Square1/1, Demux5/1, Demux6/1, Demux7/1, Square2/1
  Vector Concatenate/1 -> Reshape (9) to [3x3] column-major/1
  Square/1 -> Demux/1
  Demux/3 -> Sum/3
  Demux/4 -> Sum/4
  Demux/2 -> Sum/2
  Demux/1 -> Sum/1
  Sum/1 -> Vector Concatenate/1
  Demux1/2 -> Product/1
  Demux1/3 -> Product/2
  Demux1/1 -> Product1/1
  Demux1/4 -> Product1/2
  Product/1 -> Sum1/1
  Product1/1 -> Sum1/2
  Sum1/1 -> Gain/1
  Gain/1 -> Vector Concatenate/2
  Demux2/2 -> Product2/1
  Demux2/4 -> Product2/2
  Demux2/1 -> Product3/1
  Demux2/3 -> Product3/2
  Product3/1 -> Sum2/2
  Product2/1 -> Sum2/1
  Sum2/1 -> Gain1/1
  Gain1/1 -> Vector Concatenate/3
  Demux3/1 -> Product5/1
  Product5/1 -> Sum3/2
  Demux3/2 -> Product4/1
  Product4/1 -> Sum3/1
  Demux3/3 -> Product4/2
  Demux3/4 -> Product5/2
  Sum3/1 -> Gain2/1
  Gain2/1 -> Vector Concatenate/4
  Demux4/3 -> Sum4/3
  Demux4/1 -> Sum4/1
  Demux4/4 -> Sum4/4
  Sum4/1 -> Vector Concatenate/5
  Demux4/2 -> Sum4/2
  Square1/1 -> Demux4/1
  Product7/1 -> Sum5/2
  Product6/1 -> Sum5/1
  Sum5/1 -> Gain3/1
  Demux5/3 -> Product7/1
  Demux5/4 -> Product7/2
  Demux5/1 -> Product6/1
  Demux5/2 -> Product6/2
  Gain3/1 -> Vector Concatenate/6
  Sum6/1 -> Gain4/1
  Demux6/2 -> Product8/1
  Gain4/1 -> Vector Concatenate/7
  Demux6/4 -> Product8/2
  Demux6/3 -> Product9/2
  Demux6/1 -> Product9/1
  Product9/1 -> Sum6/2
  Product8/1 -> Sum6/1
  Demux7/2 -> Product10/2
  Demux7/3 -> Product11/1
  Sum7/1 -> Gain5/1
  Product10/1 -> Sum7/1
  Demux7/1 -> Product10/1
  Demux7/4 -> Product11/2
  Product11/1 -> Sum7/2
  Gain5/1 -> Vector Concatenate/8
  Demux8/2 -> Sum8/2
  Square2/1 -> Demux8/1
  Sum8/1 -> Vector Concatenate/9
  Demux8/3 -> Sum8/3
  Reshape (9) to [3x3] column-major/1 -> DCM/1
  Demux8/1 -> Sum8/1
  Demux8/4 -> Sum8/4

== system modelR2020a/S//C DYNAMICS (ATTITUDE + ORBIT PROPAGATION)/Orbit perturbations ==
  "[r;v]" : Inport
  Constant : Constant  Value=settings.orbitPert.J2
  If : If  IfExpression=u1
  J2 perturbation : Subsystem
  Terminator : Terminator
  if J2 perturbation : Subsystem  TreatAsAtomicUnit=on
  p : Outport
  wires:
  "[r;v]"/1 -> if J2 perturbation/1("[r;v]1")
  if J2 perturbation/1(Out1) -> J2 perturbation/1("[r;v]")
  J2 perturbation/1(p) -> p/1
  Constant/1 -> If/1
  If/2 -> Terminator/1
  If/1 -> if J2 perturbation/Action

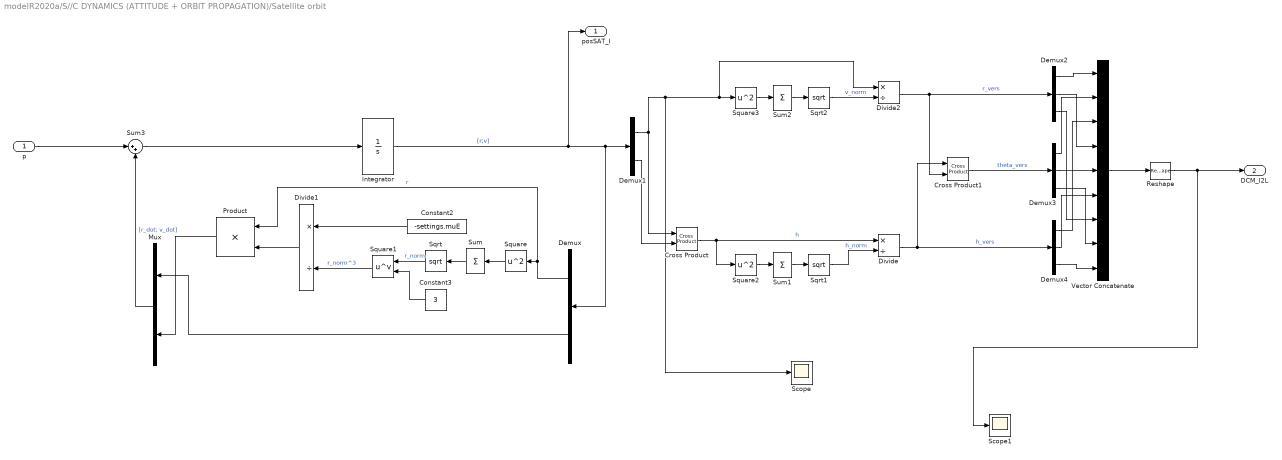
== system modelR2020a/S//C DYNAMICS (ATTITUDE + ORBIT PROPAGATION)/Satellite orbit ==
  p : Inport
  Constant2 : Constant  Value=-settings.muE
  Constant3 : Constant  Value=3
  Cross Product : vrlib/Utilities/Cross Product
  Cross Product1 : vrlib/Utilities/Cross Product
  Demux : Demux  Outputs=2
  Demux1 : Demux  Outputs=2
  Demux2 : Demux  Outputs=3
  Demux3 : Demux  Outputs=3
  Demux4 : Demux  Outputs=3
  Divide : Product  Inputs=*/
  Divide1 : Product  Inputs=*/
  Divide2 : Product  Inputs=*/
  Integrator : Integrator  InitialCondition=settings.Y0
  Mux : Mux  Inputs=2
  Product : Product
  Reshape : Reshape  OutputDimensionality=Customize  OutputDimensions=[3,3]
  Scope : Scope
  Scope1 : Scope
  Sqrt : Sqrt  SaturateOnIntegerOverflow=on
  Sqrt1 : Sqrt  SaturateOnIntegerOverflow=on
  Sqrt2 : Sqrt  SaturateOnIntegerOverflow=on
  Square : Math  Operator=square  SaturateOnIntegerOverflow=on
  Square1 : Math  Operator=pow  SaturateOnIntegerOverflow=on
  Square2 : Math  Operator=square  SaturateOnIntegerOverflow=on
  Square3 : Math  Operator=square  SaturateOnIntegerOverflow=on
  Sum : Sum  Inputs=+
  Sum1 : Sum  Inputs=+
  Sum2 : Sum  Inputs=+
  Sum3 : Sum  Inputs=|++
  Vector Concatenate : Concatenate  NumInputs=9
  posSAT_I : Outport
  DCM_I2L : Outport  Port=2
  wires:
  Constant3/1 -> Square1/2
  Demux/1 -> Product/1, Square/1  "r"
  Demux/2 -> Mux/1
  Integrator/1 -> Demux1/1, Demux/1, posSAT_I/1  "[r;v]"
  Divide1/1 -> Product/2
  Sqrt/1 -> Square1/1  "r_norm"
  Constant2/1 -> Divide1/1
  Product/1 -> Mux/2
  Sum/1 -> Sqrt/1
  Square/1 -> Sum/1
  Square1/1 -> Divide1/2  "r_norm^3"
  Mux/1 -> Sum3/2  "[r_dot; v_dot]"
  Sqrt2/1 -> Divide2/2  "v_norm"
  Divide2/1 -> Cross Product1/2, Demux2/1  "r_vers"
  Demux1/1 -> Cross Product/1, Scope/1, Divide2/1, Square3/1
  Demux2/2 -> Vector Concatenate/4
  Sqrt1/1 -> Divide/2  "h_norm"
  Demux4/1 -> Vector Concatenate/3
  Demux4/3 -> Vector Concatenate/9
  Demux3/3 -> Vector Concatenate/8
  Demux4/2 -> Vector Concatenate/6
  Vector Concatenate/1 -> Reshape/1
  Divide/1 -> Cross Product1/1, Demux4/1  "h_vers"
  Demux3/1 -> Vector Concatenate/2
  Sum1/1 -> Sqrt1/1
  Demux2/3 -> Vector Concatenate/7
  Square2/1 -> Sum1/1
  Demux2/1 -> Vector Concatenate/1
  Demux3/2 -> Vector Concatenate/5
  Cross Product/1 -> Divide/1, Square2/1  "h"
  Square3/1 -> Sum2/1
  Sum2/1 -> Sqrt2/1
  Cross Product1/1 -> Demux3/1  "theta_vers"
  Reshape/1 -> Scope1/1, DCM_I2L/1
  Demux1/2 -> Cross Product/2
  Sum3/1 -> Integrator/1
  p/1 -> Sum3/1

== system modelR2020a/SENSORS/Gyroscope ==
  omega : Inport
  ARW : RandomNumber  Variance=(1/4*deg2rad(settings.GyroscopeARW*[1;1;1]/sqrt(3600))).^2  Seed=1  SampleTime=1/settings.GyroscopeSampleRate
  Integrator : Integrator
  Integrator1 : Integrator  InitialCondition=[0 0 0 0 0 0]'
  MATLAB Function : MATLAB Function  TreatAsAtomicUnit=on
  MATLAB Function1 : MATLAB Function  TreatAsAtomicUnit=on
  RRW : RandomNumber  Variance=(1/4*deg2rad(settings.GyroscopeRRW*[1;1;1]/3600^3)).^2  Seed=2  SampleTime=1/settings.GyroscopeSampleRate
  Sum : Sum  Inputs=+++
  omega_sens : Outport
  wires:
  Sum/1 -> MATLAB Function/2(om)
  RRW/1 -> Integrator/1
  ARW/1 -> Sum/2
  Integrator/1 -> Sum/3
  omega/1 -> Sum/1
  MATLAB Function/1(x_dot) -> Integrator1/1
  Integrator1/1 -> MATLAB Function1/1(state_vector), MATLAB Function/1(x)
  MATLAB Function1/1(omega_raw) -> omega_sens/1

== system modelR2020a/SENSORS/If Action Subsystem ==
  v_B2 : Inport
  Action Port : ActionPort  ActionPortLabel=if(u1 < 1)
  Data Store Write : DataStoreWrite  DataStoreName=val
  wires:
  v_B2/1 -> Data Store Write/1

== system modelR2020a/SENSORS/If Action Subsystem1 ==
  AperA : Inport
  Action Port : ActionPort  ActionPortLabel=if(u1 < 1)
  Data Store Write : DataStoreWrite  DataStoreName=val1
  wires:
  AperA/1 -> Data Store Write/1

== system modelR2020a/SENSORS/Subsystem ==
  Earth Horizon : Constant  Value=settings.EarthSensorAccuracy
  MATLAB Function7 : MATLAB Function  TreatAsAtomicUnit=on
  Sun Sensor : Constant  Value=settings.SunSensorAccuracy
  err_EH : RandomNumber  Variance=(1/4*deg2rad(settings.EarthSensorAccuracy*[1 1 1])).^2  Seed=[1 2 3]  SampleTime=1/settings.EarthSensorSampleRate
  err_SS : RandomNumber  Variance=(1/4*deg2rad(settings.SunSensorAccuracy*[1 1 1])).^2  Seed=[4 5 6]  SampleTime=1/settings.SunSensorSampleRate
  accuracy_sens1 : Outport
  accuracy_sens2 : Outport  Port=2
  A_epsilon1 : Outport  Port=3
  A_epsilon2 : Outport  Port=4
  wires:
  MATLAB Function7/1(A_epsilon1) -> A_epsilon1/1
  MATLAB Function7/2(A_epsilon2) -> A_epsilon2/1
  Earth Horizon/1 -> accuracy_sens1/1
  Sun Sensor/1 -> accuracy_sens2/1
  err_SS/1 -> MATLAB Function7/2(accuracy_sens2)
  err_EH/1 -> MATLAB Function7/1(accuracy_sens1)

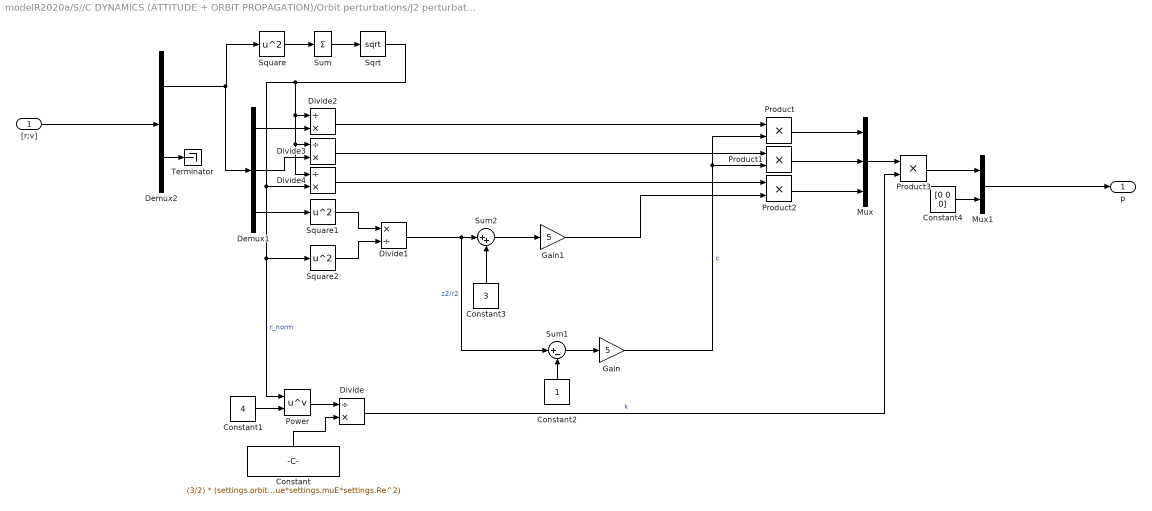
== system modelR2020a/S//C DYNAMICS (ATTITUDE + ORBIT PROPAGATION)/Orbit perturbations/J2 perturbation ==
  "[r;v]" : Inport
  Constant : Constant  Value=(3/2) * (settings.orbitPert.J2value*settings.muE*settings.Re^2)
  Constant1 : Constant  Value=4
  Constant2 : Constant
  Constant3 : Constant  Value=3
  Constant4 : Constant  Value=[0 0 0]
  Demux1 : Demux  Outputs=3
  Demux2 : Demux  Outputs=2
  Divide{,2..4} (4 alike) : Product  Inputs=/*
  Divide1 : Product  Inputs=*/
  Gain : Gain  Gain=5
  Gain1 : Gain  Gain=5
  Mux : Mux  Inputs=3
  Mux1 : Mux  Inputs=2
  Power : Math  Operator=pow  SaturateOnIntegerOverflow=on
  Product{,1..3} (4 alike) : Product
  Sqrt : Sqrt  SaturateOnIntegerOverflow=on
  Square : Math  Operator=square  SaturateOnIntegerOverflow=on
  Square1 : Math  Operator=square  SaturateOnIntegerOverflow=on
  Square2 : Math  Operator=square  SaturateOnIntegerOverflow=on
  Sum : Sum  Inputs=+
  Sum1 : Sum  Inputs=|+-
  Sum2 : Sum  Inputs=|++
  Terminator : Terminator
  p : Outport
  wires:
  "[r;v]"/1 -> Demux2/1
  Demux2/2 -> Terminator/1
  Square/1 -> Sum/1
  Sum/1 -> Sqrt/1
  Sqrt/1 -> Divide4/1, Divide3/1, Divide2/1, Divide4/2, Power/1, Square2/1  "r_norm"
  Demux2/1 -> Demux1/1, Square/1
  Constant/1 -> Divide/2
  Constant1/1 -> Power/2
  Power/1 -> Divide/1
  Demux1/3 -> Square1/1
  Square1/1 -> Divide1/1
  Square2/1 -> Divide1/2
  Constant2/1 -> Sum1/2
  Divide1/1 -> Sum1/1, Sum2/1  "z2/r2"
  Sum1/1 -> Gain/1
  Gain/1 -> Product1/2, Product/2  "c"
  Divide/1 -> Product3/2  "k"
  Demux1/1 -> Divide2/2
  Divide2/1 -> Product/1
  Demux1/2 -> Divide3/2
  Divide3/1 -> Product1/1
  Constant3/1 -> Sum2/2
  Sum2/1 -> Gain1/1
  Divide4/1 -> Product2/1
  Gain1/1 -> Product2/2
  Product/1 -> Mux/1
  Product1/1 -> Mux/2
  Product2/1 -> Mux/3
  Mux/1 -> Product3/1
  Product3/1 -> Mux1/1
  Constant4/1 -> Mux1/2
  Mux1/1 -> p/1

== system modelR2020a/S//C DYNAMICS (ATTITUDE + ORBIT PROPAGATION)/Orbit perturbations/if J2 perturbation ==
  "[r;v]1" : Inport
  Action Port : ActionPort  ActionPortLabel=if(u1)
  Out1 : Outport
  wires:
  "[r;v]1"/1 -> Out1/1

== matlab function modelR2020a/CONTROL AND ACTUATORS/MATLAB Function2 ==
  data: MagMax input; B_sensed input; Mc input; D output; M_eff_sensed output
function [D, M_eff_sensed] = fcn(MagMax,B_sensed,Mc)
D = cross(B_sensed, Mc)/norm(B_sensed);
if D(1)>MagMax
    D(1)=MagMax;
end
if D(2)>MagMax
    D(2)=MagMax;
end
if D(3)>MagMax
    D(3)=MagMax;
end
if D(1)<-MagMax
    D(1)=-MagMax;
end
if D(2)<-MagMax
    D(2)=-MagMax;
end
if D(3)<-MagMax
    D(3)=-MagMax;
end
M_eff_sensed=cross(D,B_sensed);

== matlab function modelR2020a/CONTROL AND ACTUATORS/If Action Subsystem/MATLAB Function ==
  data: rv input; w_e output; A_BI_sensed input; A_LI input; estW input; A_e output; A_BI input; pointing_err output
function [w_e, A_e, pointing_err]  = fcn(rv, A_BI_sensed, A_LI, estW, A_BI)
r = rv(1:3,1);
v = rv(4:6,1);

%% Calculating Target Attitude Matrix
X_B  = A_LI'*[-1;0;0];    % Inertial position of Earth
h_vers = cross(r,v)/norm(cross(r,v));
r_vers = r/norm(r);
trasversal_velocity_vers = cross(h_vers, r_vers);
Y_B = -trasversal_velocity_vers;
Z_B = cross(X_B,Y_B);

A_T = [X_B';Y_B';Z_B'];
A_e = A_BI_sensed*A_T';

w_target = cross(r,v)/(norm(r)^2);

w_e = estW - A_e*w_target;

X_B_actual = A_BI'*[1;0;0];
pointing_err = rad2deg(acos(dot(X_B,X_B_actual)));

== matlab function modelR2020a/CONTROL AND ACTUATORS/If Action Subsystem3/MATLAB Function ==
  data: rv input; w_e output; A_BI_sensed input; A_LI input; estW input; A_e output; A_BI input; pointing_err output
function [w_e, A_e, pointing_err]  = fcn(rv, A_BI_sensed, A_LI, estW, A_BI)
r = rv(1:3,1);
v = rv(4:6,1);

%% Calculating Target Attitude Matrix
X_B  = A_LI'*[-1;0;0];    % Inertial position of Earth
h_vers = cross(r,v)/norm(cross(r,v));
r_vers = r/norm(r);
trasversal_velocity_vers = cross(h_vers, r_vers);
Y_B = -trasversal_velocity_vers;
Z_B = cross(X_B,Y_B);

A_T = [X_B';Y_B';Z_B'];
A_e = A_BI_sensed*A_T';

w_target = cross(r,v)/(norm(r)^2);

w_e = estW - A_e*w_target;

X_B_actual = A_BI'*[1;0;0];
pointing_err = rad2deg(acos(dot(X_B,X_B_actual)));

== matlab function modelR2020a/CONTROL AND ACTUATORS/If Action Subsystem3/MATLAB Function1 ==
  data: w_e input; Mc output; A_e input; estW input; estMD input; k1 input; k2 input; J input
function Mc = fcn(w_e, A_e, estW, estMD, k1, k2, J)

AeT_AeV = [A_e(2,3) - A_e(3,2), A_e(3,1) - A_e(1,3), A_e(1,2) - A_e(2,1)]';

Mc = -k1*w_e - k2*AeT_AeV + cross(estW, J*estW) - estMD;

== matlab function modelR2020a/CONTROL AND ACTUATORS/Actual Torque produced by RW1 ==
  data: dwr input; MeffRW output; wr input; w input; Irw input
function MeffRW = fcn(dwr,wr,w,Irw)

A=[1 0 0; 0 1 0; 0 0 1];
Irw=Irw*eye(3);
hr=Irw*wr;
dhr=Irw*dwr;
MeffRW=-A*dhr-cross(w,A*hr);

== matlab function modelR2020a/CONTROL AND ACTUATORS/MATLAB Function3 ==
  data: Mc input; w_b_sensed input; dwr output; Irw input; wr input
function dwr = fcn(Mc,w_b_sensed,Irw,wr)

A=[1 0 0; 0 1 0; 0 0 1];

Irwmat = Irw*eye(3);
hr = Irwmat*wr;
F = cross(A*hr,w_b_sensed)-Mc;
G = A\F;
dhr = G(1:3,1);
dwr = dhr/Irw;

== matlab function modelR2020a/SENSORS/MATLAB Function12 ==
  data: A_BN input; A_BN_sens output; S_N input; rv input; A_BN_estim input; isEclipse input; last_v_B2 input; lastAperA input; accuracy_sens1 input; accuracy_sens2 input; A_epsilon1 input; A_epsilon2 input; v_B2 output; AperA output
function [A_BN_sens, v_B2, AperA]  = sensorModel(A_BN, S_N, rv, A_BN_estim, isEclipse, last_v_B2, lastAperA, accuracy_sens1, accuracy_sens2, A_epsilon1, A_epsilon2)

r_N = rv(1:3, 1)/norm(rv(1:3, 1)); % unit vector that identifies S/C's position w.r.t.
                            % inertial frame centered at Earth
                            
S_N = S_N / norm(S_N);  % unit vector that identifies Sun direction in the
                        % inertial frame
v_N1 = r_N;     v_N2 = S_N;



v_B1 = A_epsilon1 * A_BN * v_N1;

v_B2 = A_epsilon2 * A_BN * v_N2;
AperA = A_epsilon2 * A_BN;
    
if isEclipse
    v_N2 = lastAperA' * last_v_B2;
    v_B2 = A_BN_estim * v_N2;
end
          


%% SVD algorithm for attitude estimation
prec_sens1 = 1/norm(accuracy_sens1);
prec_sens2 = 1/norm(accuracy_sens2);
if isEclipse
    prec_sens2 = 0.001*prec_sens2;
end
alpha = [prec_sens1 prec_sens2] / (prec_sens1+prec_sens2); % s.t. sum(alpha) = 1


B = alpha(1)*v_B1*v_N1' + alpha(2)*v_B2*v_N2';

[U,~,V] = svd(B);
M = diag([1, 1, det(U)*det(V)]);
A_BN_sens = U*M*V';

== matlab function modelR2020a/SENSORS/MATLAB Function13 ==
  data: A_est input; A_raw input; w input; y output; alpha1 input
function y = stateObserbver(A_est, A_raw, w, alpha1)


W = [0,    -w(3),  w(2);
     w(3),   0,   -w(1);
    -w(2),  w(1),   0];


A_est_dot = -W * A_est + alpha1*(A_est-A_raw);


y = A_est_dot;

== matlab function modelR2020a/SENSORS/MATLAB Function2 ==
  data: A input; y output
function y = orthonorm(A)

% Recall: for a matrix to be orthonormal it is necessary that
%         det(A)=1  -->  tr(A'A - I) = 0

tol = 1e-7;
k = 0;
while trace(A'*A - eye(3,3)) > tol
    k = k+1;
    A = 3/2 * A - 1/2 * A*A'*A;
end

y = A;

== matlab function modelR2020a/SENSORS/Subsystem/MATLAB Function7 ==
  data: accuracy_sens1 input; A_epsilon1 output; accuracy_sens2 input; A_epsilon2 output
function [A_epsilon1, A_epsilon2] = sensor_error(accuracy_sens1, accuracy_sens2)


psi_acc = accuracy_sens1(1);
th_acc  = accuracy_sens1(2);
phi_acc = accuracy_sens1(3);
A_epsilon1 = [cos(psi_acc)*cos(th_acc)  (cos(psi_acc)*sin(th_acc)*sin(phi_acc)+sin(psi_acc)*cos(phi_acc)) (-cos(psi_acc)*sin(th_acc)*cos(phi_acc)+sin(psi_acc)*sin(phi_acc));
                -sin(psi_acc)*cos(th_acc) (-sin(psi_acc)*sin(th_acc)*sin(phi_acc)+cos(psi_acc)*cos(phi_acc))  (sin(psi_acc)*sin(th_acc)*cos(phi_acc)+cos(psi_acc)*sin(phi_acc));
                 sin(th_acc)               -cos(th_acc)*sin(phi_acc)                                           cos(th_acc)*cos(phi_acc)];
             
             

psi_acc = accuracy_sens2(1);
th_acc  = accuracy_sens2(2);
phi_acc = accuracy_sens2(3);
A_epsilon2 = [cos(psi_acc)*cos(th_acc)  (cos(psi_acc)*sin(th_acc)*sin(phi_acc)+sin(psi_acc)*cos(phi_acc)) (-cos(psi_acc)*sin(th_acc)*cos(phi_acc)+sin(psi_acc)*sin(phi_acc));
                -sin(psi_acc)*cos(th_acc) (-sin(psi_acc)*sin(th_acc)*sin(phi_acc)+cos(psi_acc)*cos(phi_acc))  (sin(psi_acc)*sin(th_acc)*cos(phi_acc)+cos(psi_acc)*sin(phi_acc));
                 sin(th_acc)               -cos(th_acc)*sin(phi_acc)                                           cos(th_acc)*cos(phi_acc)];


end

== matlab function modelR2020a/S//C DYNAMICS (ATTITUDE + ORBIT PROPAGATION)/disturbanceTorques ==
  data: J input; M_disturbance output; r_CG input; A_BN input; A_BL input; S_B input; rr input; vv input; C_D input; rho input; t input; b_B output; isEclipse output; gamma output
function [M_disturbance, b_B, isEclipse, gamma] = disturbanceTorquesa(J, r_CG, A_BN, A_BL, S_B, rr, vv, C_D, rho, t)



G = 6.67408e-11;
m_E = 5.972e+24;
kep = car2par(rr, vv, 398600);
a = kep(1); e = kep(2); i = kep(3);
OM = kep(4); om = kep(5); th = kep(6);
R_equat = 6371e+3; % [m]
p = a*(1-e^2);
R = p / (1+e*cos(th)) * 1e+3; % [m]





% Moments of Inertia [kg*m^2]
% (12U Cubesat)
J1 = J(1,1);
J2 = J(2,2);
J3 = J(3,3);





C1 = (J2-J3)/J1;
C2 = (J3-J1)/J2;
C3 = (J1-J2)/J3;






%% Gravity Gradient Torque
c = A_BL * [1;0;0];



M_GG = [- 3*G*m_E/R^3 *C1* c(3)*c(2);
- 3*G*m_E/R^3 *C2* c(1)*c(3);
- 3*G*m_E/R^3 *C3* c(2)*c(1)];



%% SRP Torque @ 600 Km (Direct Solar Rad. + Sun Rad. Reflected by Earth + Earth Rad.)
isEclipse = 0;
S_I = A_BN'*S_B;
S_Iv = S_I/norm(S_I);
rrv = rr/norm(rr);
gamma = acos(dot(rrv,-S_Iv));
gamma_max = atan((R_equat/1000)/norm(rr));

if abs(gamma) <= gamma_max
    F_e = 143.4; % [W/m^2]
    isEclipse = 1;
else
    F_e = 1358 + 580 + 143.4; % [W/m^2]
end

P = F_e / (3*1e+8);



N_body = 6; % # main body surfaces
N_SP = 4; % # solar panel surfaces



U = 0.1; % 1U length



N = zeros(N_body+N_SP,3);
A = zeros(N_body+N_SP,1);
r = zeros(N_body+N_SP,3);
n1 = [1 0 0]; n2 = [0 1 0]; n3 = [0 0 1];
% S/C Main Body: Normals, Surface Coefficients, Areas
N(1,:) = n1; N(2,:) = n2; N(3,:) = n3;
N(4,:) = -n1; N(5,:) = -n2; N(6,:) = -n3;
rho_s_body = 0.6; rho_d_body = 0.1;
A(1:N_body) = [4 6 6 4 6 6]*U^2; % [m^2]



% Solar Panels: Normals, Surface Coefficients, Areas
N(7,:) = n1; N(8,:) = -n1; N(9,:) = n1; N(10,:) = -n1;
rho_s_SP = 0.6; rho_d_SP = 0.1;
A(N_body+1:N_body+N_SP) = [12 12 12 12]*U^2; % [m^2]



% L.u.c. a RF centered @ Geometric Center of S/C::
% we will use it to define the coordinates of each surface's center
% along w/ the coordinates of th CG w.r.t. GC
r(1,:) = [1.5 0 0]*U; r(2,:) = [0 1 0]*U; r(3,:) = [0 0 1]*U;
r(4,:) = [-1.5 0 0]*U; r(5,:) = [0 -1 0]*U; r(6,:) = [0 0 -1]*U;
r(7,:) = [0 5 0]*U; r(8,:) = [0 5 0]*U;
r(9,:) = [0 -5 0]*U; r(10,:) = [0 -5 0]*U;



S_B_norm = S_B / norm(S_B);



M_SRP = zeros(3,1);
for k = 1:N_body+N_SP
if k <= N_body
rho_s = rho_s_body; rho_d = rho_d_body;
else
rho_s = rho_s_SP; rho_d = rho_d_SP;
end



n_k = N(k,:)';
F_k = - P*A(k)*dot(S_B_norm,n_k) * ( (1-rho_s)*S_B_norm + (2*rho_s*dot(S_B_norm,n_k)+2/3*rho_d)*n_k );



if dot(S_B_norm, n_k) > 0
r_k = (r(k,:) - r_CG')';
M_SRP_k = cross(r_k, F_k);
else
M_SRP_k = zeros(3,1);
end



M_SRP = M_SRP + M_SRP_k;



end




%% Air-Drag Torque
w_E = 2*pi/(23*3600 + 56*60 + 4.09); % Earth's angular rate [rad/s]
mu_E = 398600.433; % [km^3/s^2]



% Rotation matrices: Earth-Centered Inertial --> Perifocal (ECI->PF)
R_om = [cos(om) sin(om) 0 ;
-sin(om) cos(om) 0 ;
0 0 1 ];



R_i = [ 1 0 0 ;
0 cos(i) sin(i);
0 -sin(i) cos(i)];



R_OM = [cos(OM) sin(OM) 0 ;
-sin(OM) cos(OM) 0 ;
0 0 1 ];



R313 = R_om * R_i * R_OM; % ECI --> PF



R_PF = R * [cos(th), sin(th), 0]';
v_PF = sqrt(mu_E/p) * [-sin(th), (e+cos(th)), 0]';
% PF --> ECI
r_ECI = R313'* R_PF;
v_ECI = R313'* v_PF;



v_rel_N = v_ECI + cross([0 0 w_E]', r_ECI);
v_rel_B = A_BN*v_rel_N; % Relative atmosphere velocity (@body frame)
v_rel_B_unit = v_rel_B / norm(v_rel_B);



M_drag = zeros(3,1);
for k = 1:N_body+N_SP



n_k = N(k,:)';
F_k = - .5 * C_D * rho * norm(v_rel_B)^2 * dot(n_k,v_rel_B_unit) * A(k) * v_rel_B_unit;



if dot(S_B_norm, n_k) > 0
r_k = (r(k,:) - r_CG')';
M_drag_k = cross(r_k, F_k);
else
M_drag_k = zeros(3,1);
end



M_drag = M_drag + M_drag_k;



end

M_drag(isnan(M_drag)) = 0;



%% Magnetic Torque
g10 = -29615e-9; g11 = -1728e-9; h11 = 5186e-9;
H0 = sqrt(g10^2 + g11^2 + h11^2);
m = [sind(11.5)*cos(w_E*t);
sind(11.5)*sin(w_E*t);
cosd(11.5)];
r_N = R * [cos(th);
sin(th)*cos(i);
sin(th)*sin(i)];



% Magnetic field vector
b_N = R_equat^3*H0/R^3 * (3*dot(m/norm(m),r_N/norm(r_N))*r_N/norm(r_N) - m/norm(m));
b_B = A_BN * b_N;
% Parasitic magnetic torque



M_magn = cross(m, b_B);
M_disturbance = [M_drag(:), M_SRP(:), M_magn(:), M_GG(:)];

== matlab function modelR2020a/CONTROL AND ACTUATORS/If Action Subsystem2/MATLAB Function ==
  data: rv input; w_e output; A_BI_sensed input; A_LI input; estW input; A_e output; A_BI input; pointing_err output
function [w_e, A_e, pointing_err]  = fcn(rv, A_BI_sensed, A_LI, estW, A_BI)
r = rv(1:3,1);
v = rv(4:6,1);

%% Calculating Target Attitude Matrix
X_B  = A_LI'*[-1;0;0];    % Inertial position of Earth
h_vers = cross(r,v)/norm(cross(r,v));
r_vers = r/norm(r);
trasversal_velocity_vers = cross(h_vers, r_vers);
Y_B = -trasversal_velocity_vers;
Z_B = cross(X_B,Y_B);

A_T = [X_B';Y_B';Z_B'];
A_e = A_BI_sensed*A_T';

w_target = cross(r,v)/(norm(r)^2);

w_e = estW - A_e*w_target;

X_B_actual = A_BI'*[1;0;0];
pointing_err = rad2deg(acos(dot(X_B,X_B_actual)));

== matlab function modelR2020a/CONTROL AND ACTUATORS/If Action Subsystem2/MATLAB Function1 ==
  data: w_e input; Mc output; A_e input; estW input; estMD input; k1 input; k2 input; J input
function Mc = fcn(w_e, A_e, estW, estMD, k1, k2, J)

AeT_AeV = [A_e(2,3) - A_e(3,2), A_e(3,1) - A_e(1,3), A_e(1,2) - A_e(2,1)]';

Mc = -k1*w_e - k2*AeT_AeV + cross(estW, J*estW) - estMD;

== matlab function modelR2020a/SENSORS/Gyroscope/MATLAB Function ==
  data: x input; x_dot output; om input; M output
function [x_dot,M] = GyroModel(x,om)
%gyro inertia parameters
Ir = 1e-7;
Jz = 2e-7;
%tuning parameter for visco-elastic reaction torque
k=10;
%tuning law for c for fastest convergence
c_gyro = 2*sqrt(k*Jz);
om_x = om(1);
om_y = om(2);
om_z = om(3);
%angular velocity of gyro wheel (100 deg/s)
om_r = 100*pi/180;



% defining the theta_i and \dot theta_i
x_dot = zeros(6,1);



th_x = x(1);
th_y = x(2);
th_z = x(3);
va_x = x(4);
va_y = x(5);
va_z = x(6);
%3 gyro dynamics expressed as 1st order differential equation
x_dot(1) = va_x;
x_dot(2) = va_y;
x_dot(3) = va_z;
x_dot(4) = -(c_gyro/Jz)*va_x-(k/Jz)*th_x-(Ir/Jz)*om_r*om_x;
x_dot(5) = -(c_gyro/Jz)*va_y-(k/Jz)*th_y-(Ir/Jz)*om_r*om_y;
x_dot(6) = -(c_gyro/Jz)*va_z-(k/Jz)*th_z-(Ir/Jz)*om_r*om_z;
%gyro outputs
x_dot=[x_dot(1) x_dot(2) x_dot(3) x_dot(4) x_dot(5) x_dot(6)]';



%feedback torque applied to the gyros
M_x = -k*th_x-c_gyro*va_x;
M_y = -k*th_y-c_gyro*va_y;
M_z = -k*th_z-c_gyro*va_z;



M = [M_x M_y M_z]';




end

== matlab function modelR2020a/SENSORS/Gyroscope/MATLAB Function1 ==
  data: state_vector input; omega_raw output
function omega_raw = fcn(state_vector)



theta_vec = state_vector(1:3);
Ir = 1e-7;
k = 10;
om_r = 100*pi/180;



omega_raw = - k*theta_vec / (Ir*om_r);



end

== matlab function modelR2020a/CONTROL AND ACTUATORS/If Action Subsystem1/MATLAB Function ==
  data: rv input; w_e output; A_BI_sensed input; A_LI input; estW input; A_e output; A_BI input; pointing_err output
function [w_e, A_e, pointing_err]  = fcn(rv, A_BI_sensed, A_LI, estW, A_BI)
r = rv(1:3,1);
v = rv(4:6,1);

%% Calculating Target Attitude Matrix
X_B  = A_LI'*[-1;0;0];    % Inertial position of Earth
h_vers = cross(r,v)/norm(cross(r,v));
r_vers = r/norm(r);
trasversal_velocity_vers = cross(h_vers, r_vers);
Y_B = -trasversal_velocity_vers;
Z_B = cross(X_B,Y_B);

A_T = [X_B';Y_B';Z_B'];
A_e = A_BI_sensed*A_T';

w_target = cross(r,v)/(norm(r)^2);

w_e = estW - A_e*w_target;

X_B_actual = A_BI'*[1;0;0];
pointing_err = rad2deg(acos(dot(X_B,X_B_actual)));
